simulink model "TwinRotor_G1_adaptativo"  (Simulink 8.6)
settings: Solver=ode1  SolverMode=SingleTasking  StartTime=0.0  StopTime=inf  FixedStep=0.05  RelTol=1e-3
values from neighbouring files (symbols this model uses):
  Kd_tr = 0.01    [def_pid.m]
  Ki_tr = 0.01    [def_pid.m]
  Kp_tr = 0.01    [def_pid.m]
libraries: RT x1
settings Model: Creator=Tomas  LastModifiedBy=pdoren
settings DataIOCC: SignalLoggingName=sigsOut
settings OptimizationCC: ExpressionDepthLimit=128  InitFltsAndDblsToZero=on
settings DebuggingCC: SaveWithParameterizedLinksMsg=none  SignalResolutionControl=TryResolveAllWithWarning  SolverPrmCheckMsg=none  MultiTaskDSMMsg=warning  MultiTaskCondExecSysMsg=none  FcnCallInpInsideContextMsg=UseLocalSettings  StateNameClashWarn=none  StrictBusMsg=None
settings HardwareCC: TargetBitPerPointer=64  TargetLongLongMode=on  TargetIntDivRoundTo=Zero  TargetEndianess=LittleEndian  TargetWordSize=64  TargetHWDeviceType=MATLAB Host  ProdEqTarget=off
settings GRTTargetCC: TargetFcnLib=ansi_tfl_tmw.mat  GeneratePreprocessorConditionals=Use local settings

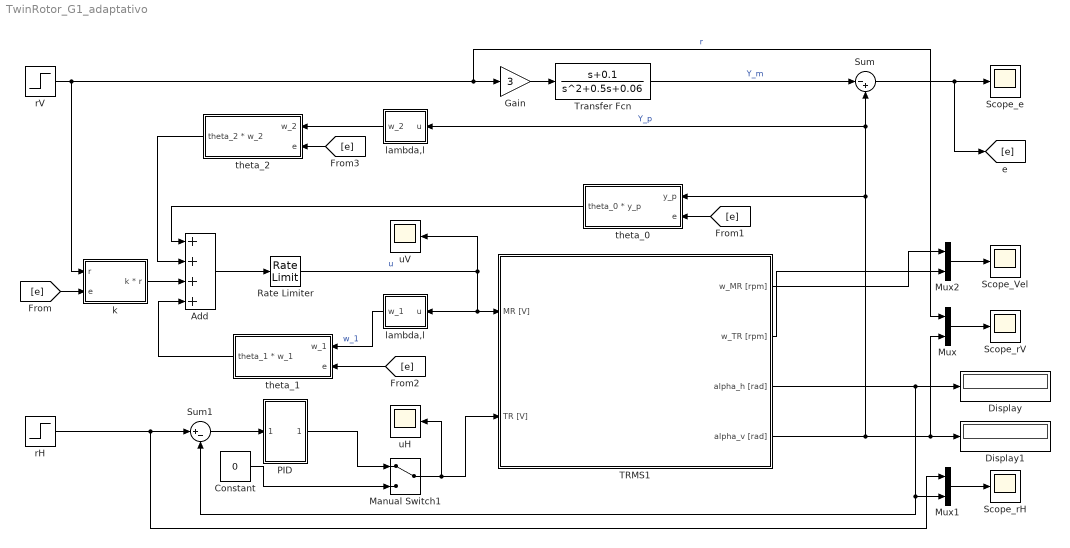
== system TwinRotor_G1_adaptativo ==
  Add : Sum  Inputs=++++
  Constant : Constant  Value=0
  Display : Display
  Display1 : Display
  Gain : Gain  Gain=3
  Manual Switch1 : ManualSwitch
  Mux : Mux  Inputs=2
  Mux1 : Mux  Inputs=2
  Mux2 : Mux  Inputs=2
  PID : Subsystem
  Rate Limiter : RateLimiter  SampleTimeMode=inherited
  Scope_Vel : Scope
  Scope_e : Scope
  Scope_rH : Scope
  Scope_rV : Scope
  Sum : Sum  Inputs=|-+
  Sum1 : Sum  Inputs=|+-
  TRMS1 : Subsystem  mask{Ts=0.05, bias_h=0, bias_v=0, max_mr=20, max_tr=15}
      mask prompts: Ts "Tiempo de Muestreo"; bias_h "bias alpha_h"; bias_v "bias alpha_v"; max_mr "voltaje MR [V]"; max_tr "voltaje TR [V]"
      mask Display:
      | image(imread('Imagenes/Copter.png'))
      | 
      | port_label('output', 1, 'w_MR [rpm]')
      | port_label('output', 2, 'w_TR [rpm]')
      | port_label('output', 3, 'alpha_h [deg]')
      | port_label('output', 4, 'alpha_v [deg]')
      | port_label('input', 1, 'MR [V]')
      | port_label('input', 2, 'TR [V]')
  Transfer Fcn : TransferFcn  Numerator=[1 0.1]  Denominator=[1 0.5 0.06]
  k : Subsystem
  lambda,l : Subsystem
  "lambda,l " : Subsystem
  rH : Step  SampleTime=0
  rV : Step  SampleTime=0
  theta_0 : Subsystem
  theta_1 : Subsystem
  theta_2 : Subsystem
  uH : Scope
  uV : Scope
  wires:
  TRMS1/4(alpha_v [rad]) -> Mux/2, Display1/1, "lambda,l "/1(u), Sum/2, theta_0/1(y_p)  "Y_p"
  TRMS1/3(alpha_h [rad]) -> Display/1, Mux1/2, Sum1/2
  PID/1(Out1) -> Manual Switch1/1
  Constant/1 -> Manual Switch1/2
  Sum1/1 -> PID/1(In1)
  Manual Switch1/1 -> uH/1, TRMS1/2(TR [V])
  rH/1 -> Sum1/1, Mux1/1
  Mux2/1 -> Scope_Vel/1
  Mux/1 -> Scope_rV/1
  Mux1/1 -> Scope_rH/1
  TRMS1/1(w_MR [rpm]) -> Mux2/1
  TRMS1/2(w_TR [rpm]) -> Mux2/2
  Gain/1 -> Transfer Fcn/1
  Sum/1 -> [e], Scope_e/1
  Transfer Fcn/1 -> Sum/1  "Y_m"
  rV/1 -> Mux/1, Gain/1, k/1(r)  "r"
  theta_0/1(theta_0 * y_p) -> Add/1
  [e] -> theta_0/2(e)
  [e] -> theta_1/2(e)
  [e] -> theta_2/2(e)
  Add/1 -> Rate Limiter/1
  Rate Limiter/1 -> lambda,l/1(u), TRMS1/1(MR [V]), uV/1  "u"
  theta_1/1(theta_1 * w_1) -> Add/4
  theta_2/1(theta_2 * w_2) -> Add/2
  lambda,l/1(w_1) -> theta_1/1(w_1)  "w_1"
  "lambda,l "/1(w_2) -> theta_2/1(w_2)
  [e] -> k/2(e)
  k/1(k * r) -> Add/3

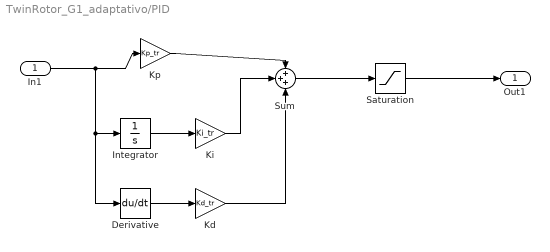
== system TwinRotor_G1_adaptativo/PID ==
  In1 : Inport
  Derivative : Derivative
  Integrator : Integrator
  Kd : Gain  Gain=Kd_tr
  Ki : Gain  Gain=Ki_tr
  Kp : Gain  Gain=Kp_tr
  Saturation : Saturate  UpperLimit=5  LowerLimit=-5
  Sum : Sum  Inputs=+++
  Out1 : Outport
  wires:
  In1/1 -> Kp/1, Integrator/1, Derivative/1
  Kp/1 -> Sum/1
  Sum/1 -> Saturation/1
  Saturation/1 -> Out1/1
  Integrator/1 -> Ki/1
  Ki/1 -> Sum/2
  Derivative/1 -> Kd/1
  Kd/1 -> Sum/3

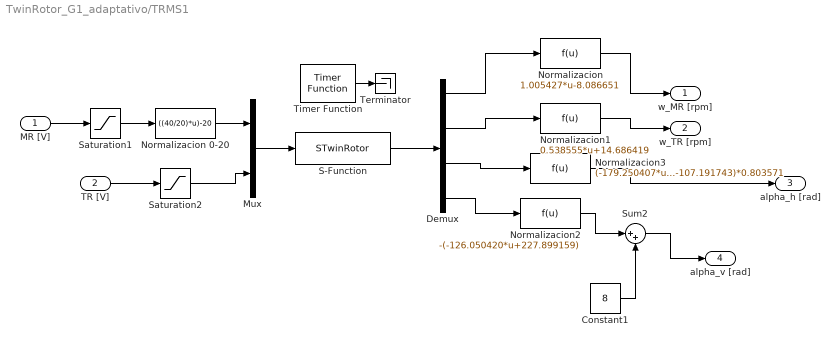
== system TwinRotor_G1_adaptativo/TRMS1 ==
  MR [V] : Inport
  TR [V] : Inport  Port=2
  Constant1 : Constant  Value=8
  Demux : Demux
  Mux : Mux  Inputs=2
  Normalizacion : Fcn  Expr=1.005427*u-8.086651
  Normalizacion 0-20 : Fcn  Expr=((40/20)*u)-20
  Normalizacion1 : Fcn  Expr=0.538555*u+14.686419
  Normalizacion2 : Fcn  Expr=-(-126.050420*u+227.899159)
  Normalizacion3 : Fcn  Expr=(-179.250407*u-107.191743)*0.803571
  S-Function : S-Function  FunctionName=STwinRotor  Parameters=Ts,bias_h,bias_v,max_mr,max_tr  SFunctionDeploymentMode=off  EnableBusSupport=off
  Saturation1 : Saturate  UpperLimit=20  LowerLimit=0
  Saturation2 : Saturate  UpperLimit=5  LowerLimit=-5
  Sum2 : Sum  Inputs=|++
  Terminator : Terminator
  Timer Function : RT/Timer Function  Priority=1234246656  step=50  ThPriority=TIME CRITICAL
  w_MR [rpm] : Outport
  w_TR [rpm] : Outport  Port=2
  alpha_h [rad] : Outport  Port=3
  alpha_v [rad] : Outport  Port=4
  wires:
  Constant1/1 -> Sum2/2
  Sum2/1 -> alpha_v [rad]/1
  Normalizacion2/1 -> Sum2/1
  Saturation2/1 -> Mux/2
  Saturation1/1 -> Normalizacion 0-20/1
  Normalizacion3/1 -> alpha_h [rad]/1
  Demux/3 -> Normalizacion3/1
  Demux/4 -> Normalizacion2/1
  Demux/2 -> Normalizacion1/1
  Normalizacion1/1 -> w_TR [rpm]/1
  Demux/1 -> Normalizacion/1
  Normalizacion/1 -> w_MR [rpm]/1
  MR [V]/1 -> Saturation1/1
  Normalizacion 0-20/1 -> Mux/1
  S-Function/1 -> Demux/1
  Mux/1 -> S-Function/1
  TR [V]/1 -> Saturation2/1
  Timer Function/1 -> Terminator/1

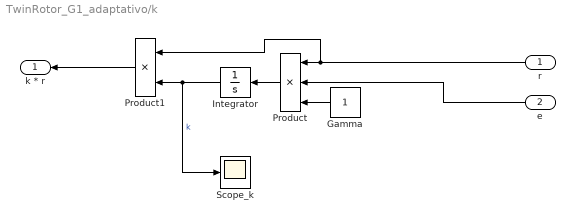
== system TwinRotor_G1_adaptativo/k ==
  r : Inport
  e : Inport  Port=2
  Gamma : Constant
  Integrator : Integrator
  Product : Product  Inputs=3
  Product1 : Product
  Scope_k : Scope
  k * r : Outport
  wires:
  r/1 -> Product1/1, Product/1
  Product1/1 -> k * r/1
  Gamma/1 -> Product/3
  Integrator/1 -> Scope_k/1, Product1/2  "k"
  Product/1 -> Integrator/1
  e/1 -> Product/2

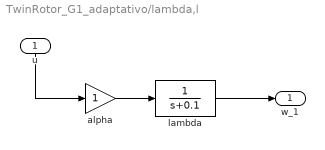
== system TwinRotor_G1_adaptativo/lambda,l ==
  u : Inport
  alpha : Gain
  lambda : TransferFcn  Denominator=[1 0.1]
  w_1 : Outport
  wires:
  alpha/1 -> lambda/1
  u/1 -> alpha/1
  lambda/1 -> w_1/1

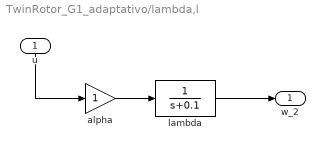
== system TwinRotor_G1_adaptativo/lambda,l  ==
  u : Inport
  alpha : Gain
  lambda : TransferFcn  Denominator=[1 0.1]
  w_2 : Outport
  wires:
  alpha/1 -> lambda/1
  u/1 -> alpha/1
  lambda/1 -> w_2/1

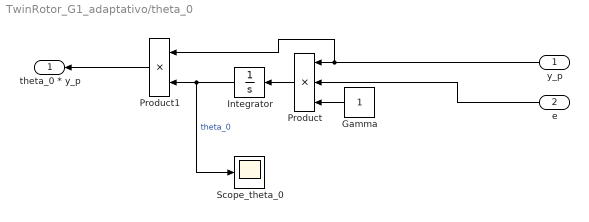
== system TwinRotor_G1_adaptativo/theta_0 ==
  y_p : Inport
  e : Inport  Port=2
  Gamma : Constant
  Integrator : Integrator
  Product : Product  Inputs=3
  Product1 : Product
  Scope_theta_0 : Scope
  theta_0 * y_p : Outport
  wires:
  y_p/1 -> Product1/1, Product/1
  Product1/1 -> theta_0 * y_p/1
  Gamma/1 -> Product/3
  Integrator/1 -> Scope_theta_0/1, Product1/2  "theta_0"
  Product/1 -> Integrator/1
  e/1 -> Product/2

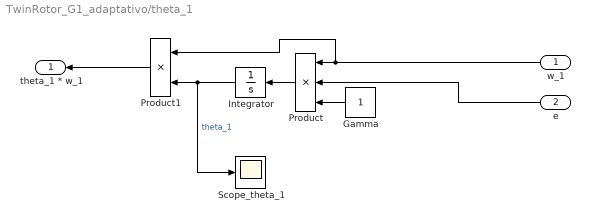
== system TwinRotor_G1_adaptativo/theta_1 ==
  w_1 : Inport
  e : Inport  Port=2
  Gamma : Constant
  Integrator : Integrator
  Product : Product  Inputs=3
  Product1 : Product
  Scope_theta_1 : Scope
  theta_1 * w_1 : Outport
  wires:
  w_1/1 -> Product1/1, Product/1
  Product1/1 -> theta_1 * w_1/1
  Gamma/1 -> Product/3
  Integrator/1 -> Scope_theta_1/1, Product1/2  "theta_1"
  Product/1 -> Integrator/1
  e/1 -> Product/2

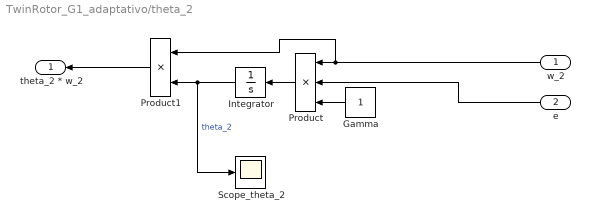
== system TwinRotor_G1_adaptativo/theta_2 ==
  w_2 : Inport
  e : Inport  Port=2
  Gamma : Constant
  Integrator : Integrator
  Product : Product  Inputs=3
  Product1 : Product
  Scope_theta_2 : Scope
  theta_2 * w_2 : Outport
  wires:
  w_2/1 -> Product1/1, Product/1
  Product1/1 -> theta_2 * w_2/1
  Gamma/1 -> Product/3
  Integrator/1 -> Scope_theta_2/1, Product1/2  "theta_2"
  Product/1 -> Integrator/1
  e/1 -> Product/2
